simulink model "simulation_base_others"  (R2013a)
settings: Solver=ode4  StartTime=0.0  StopTime=0.2  FixedStep=Ts  RelTol=1e-3
values from neighbouring files (symbols this model uses):
  Cdc = 5e-3    (= 0.005)    [rpg_simulation_base.m]
  Crpcu_each = 1/(2*pi*fs*Zrpcu_each)    [rpg_simulation_base.m]
  ESR = 1e-3    (= 0.001)    [rpg_simulation_base.m]
  fs = 50    [rpg_loss_calculation.m]    (also in rpg_simulation_base.m)
  ftr = 50    [rpg_simulation_base.m]
  Lcable = Xcable/(2*pi*fs)    (= 7.16197243914e-05)    [rpg_simulation_base.m]
  Lload = Xload/wout    [rpg_simulation_base.m]
  Lload1 = Xload1/(2*pi*fs)    [rpg_simulation_base.m]
  Lpri_pu = 0.025    [rpg_simulation_base.m]
  Ls = 1e-3    (= 0.001)    [rpg_simulation_base.m]
  Lsec_pu = 0.025    [rpg_simulation_base.m]
  Ppv = 40e3    (= 40000)    [rpg_simulation_base.m]
  Qpv = 30e3    (= 30000)    [rpg_simulation_base.m]
  Rcable = 56.4e-3    (= 0.0564)    [rpg_simulation_base.m]
  Rload = Zload*pf    [rpg_simulation_base.m]
  Rload1 = Zload1*pfload1    [rpg_simulation_base.m]
  RLs = 10e-3    (= 0.01)    [rpg_simulation_base.m]
  Rpri_pu = 0.0025    [rpg_simulation_base.m]
  Rsec_pu = 0.0025    [rpg_simulation_base.m]
  Rseries = 5    [rpg_simulation_base.m]
  Sbase = 1.6e6    (= 1600000)    [rpg_simulation_base.m]
  Ts = 1e-5    (= 1e-05)    [rpg_simulation_base.m]
  V1 = Vdc*(Rseries+Rrefl)/Rrefl    (= 1083.33333333)    [rpg_simulation_base.m]
  Vdc = 750    [calculate_loss.m]    (also in rpg_loss_calculation.m; rpg_simulation_base.m)
  Vline = 400    [calculate_loss.m]    (also in rpg_loss_calculation.m; rpg_simulation_base.m = 34500)
  Vphase = 400/sqrt(3)    [rpg_simulation_base.m]
  Vpri = 34.5e3    (= 34500)    [rpg_simulation_base.m]
  Vsec = 400    [rpg_simulation_base.m]
  Xs = 2*pi*fs*Ls    (= 0.314159265359)    [rpg_simulation_base.m]
undefined symbols (not defined in the file or in its folder): Lload2, Rload2, rpcu_s1, rpcu_s2, rpcu_s3, rpcu_s4
libraries: powerlib x107, powerlib_meascontrol x18, simulink x1
settings Model: Creator=hp  LastModifiedBy=ugurm

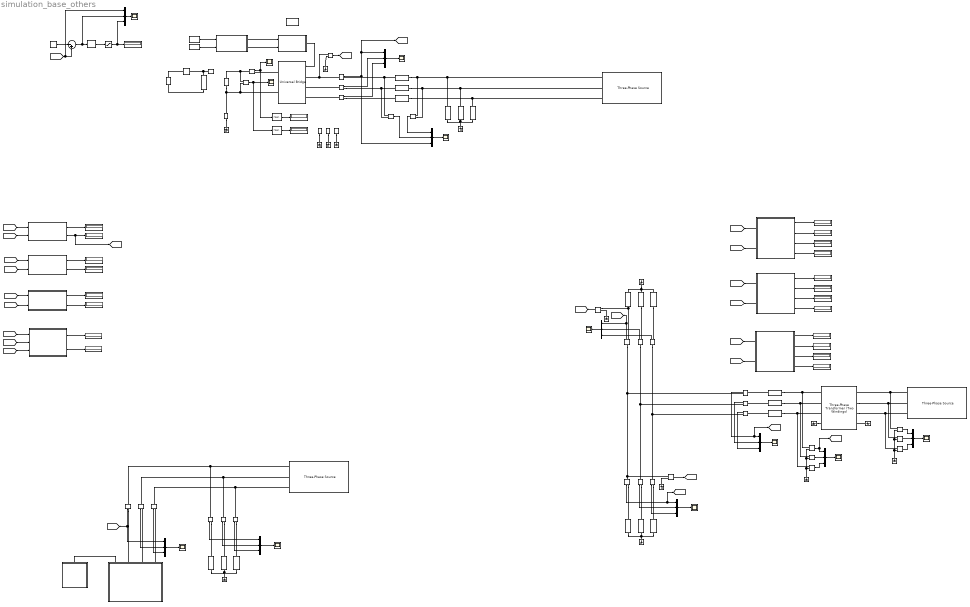
== system simulation_base_others ==
  note: LATER
  note: Grid side P and Q
  note: Load side P and Q
  note: RPCU side P and Q
  note: PV side P and Q
  note: Load-2 P&Q
  note: Load-1 P&Q
  note: PCC P&Q
  Cable_a : powerlib/Elements/Series RLC Branch  LConnTagsString=__new0  RConnTagsString=__new0  BranchType=RL  Resistance=Rcable  Inductance=Lcable  SetiL0=off  InitialCurrent=0  Capacitance=1e-6  Setx0=off  InitialVoltage=0  Measurements=None
  Cable_b : powerlib/Elements/Series RLC Branch  LConnTagsString=__new0  RConnTagsString=__new0  BranchType=RL  Resistance=Rcable  Inductance=Lcable  SetiL0=off  InitialCurrent=0  Capacitance=1e-6  Setx0=off  InitialVoltage=0  Measurements=None
  Cable_c : powerlib/Elements/Series RLC Branch  LConnTagsString=__new0  RConnTagsString=__new0  BranchType=RL  Resistance=Rcable  Inductance=Lcable  SetiL0=off  InitialCurrent=0  Capacitance=1e-6  Setx0=off  InitialVoltage=0  Measurements=None
  Compensation unit : Subsystem
  DC bus cap : powerlib/Elements/Series RLC Branch  LConnTagsString=__new0  RConnTagsString=__new0  BranchType=RC  Resistance=ESR  Inductance=1e-3  SetiL0=off  InitialCurrent=0  Capacitance=Cdc  Setx0=on  InitialVoltage=600  Measurements=None
  Filter_a : powerlib/Elements/Series RLC Branch  LConnTagsString=__new0  RConnTagsString=__new0  BranchType=RL  Resistance=RLs  Inductance=Ls  SetiL0=off  InitialCurrent=0  Capacitance=1e-6  Setx0=off  InitialVoltage=0  Measurements=None
  Filter_b : powerlib/Elements/Series RLC Branch  LConnTagsString=__new0  RConnTagsString=__new0  BranchType=RL  Resistance=RLs  Inductance=Ls  SetiL0=off  InitialCurrent=0  Capacitance=1e-6  Setx0=off  InitialVoltage=0  Measurements=None
  Filter_c : powerlib/Elements/Series RLC Branch  LConnTagsString=__new0  RConnTagsString=__new0  BranchType=RL  Resistance=RLs  Inductance=Ls  SetiL0=off  InitialCurrent=0  Capacitance=1e-6  Setx0=off  InitialVoltage=0  Measurements=None
  Grid (infinite bus) : powerlib/Electrical Sources/Three-Phase Source  Voltage=Vline  PhaseAngle=0  Frequency=fs  InternalConnection=Yg  SpecifyImpedance=off  Resistance=0  Inductance=0  ShortCircuitLevel=100e6  BaseVoltage=Vline  XRratio=7  BusType=swing  Pref=0  Qref=0  Qmin=-inf  Qmax=inf
  Grid (infinite bus)1 : powerlib/Electrical Sources/Three-Phase Source  Voltage=Vline  PhaseAngle=0  Frequency=fs  InternalConnection=Yg  SpecifyImpedance=off  Resistance=1e-9  Inductance=1e-9  ShortCircuitLevel=100e6  BaseVoltage=Vline  XRratio=7  BusType=swing  Pref=0  Qref=0  Qmin=-inf  Qmax=inf
  Grid (infinite bus)2 : powerlib/Electrical Sources/Three-Phase Source  Voltage=400  PhaseAngle=0  Frequency=fs  InternalConnection=Yg  SpecifyImpedance=off  Resistance=0  Inductance=0  ShortCircuitLevel=100e6  BaseVoltage=400  XRratio=7  BusType=swing  Pref=0  Qref=0  Qmin=-inf  Qmax=inf
  Ground{,1..14} (15 alike) : powerlib/Elements/Ground  LConnTagsString=a
  Load_1a : powerlib/Elements/Series RLC Branch  LConnTagsString=__new0  RConnTagsString=__new0  BranchType=RL  Resistance=Rload1  Inductance=Lload1  SetiL0=off  InitialCurrent=0  Capacitance=1e-6  Setx0=off  InitialVoltage=0  Measurements=None
  Load_1b : powerlib/Elements/Series RLC Branch  LConnTagsString=__new0  RConnTagsString=__new0  BranchType=RL  Resistance=Rload1  Inductance=Lload1  SetiL0=off  InitialCurrent=0  Capacitance=1e-6  Setx0=off  InitialVoltage=0  Measurements=None
  Load_1c : powerlib/Elements/Series RLC Branch  LConnTagsString=__new0  RConnTagsString=__new0  BranchType=RL  Resistance=Rload1  Inductance=Lload1  SetiL0=off  InitialCurrent=0  Capacitance=1e-6  Setx0=off  InitialVoltage=0  Measurements=None
  Load_2a : powerlib/Elements/Series RLC Branch  LConnTagsString=__new0  RConnTagsString=__new0  BranchType=RL  Resistance=Rload2  Inductance=Lload2  SetiL0=off  InitialCurrent=0  Capacitance=1e-6  Setx0=off  InitialVoltage=0  Measurements=None
  Load_2a1 : powerlib/Elements/Series RLC Branch  LConnTagsString=__new0  RConnTagsString=__new0  BranchType=RL  Resistance=Rload2  Inductance=Lload2  SetiL0=off  InitialCurrent=0  Capacitance=1e-6  Setx0=off  InitialVoltage=0  Measurements=None
  Load_2a2 : powerlib/Elements/Series RLC Branch  LConnTagsString=__new0  RConnTagsString=__new0  BranchType=RL  Resistance=Rload2  Inductance=Lload2  SetiL0=off  InitialCurrent=0  Capacitance=1e-6  Setx0=off  InitialVoltage=0  Measurements=None
  Load_a1 : powerlib/Elements/Series RLC Branch  LConnTagsString=__new0  RConnTagsString=__new0  BranchType=RL  Resistance=Rload  Inductance=Lload  SetiL0=off  InitialCurrent=0  Capacitance=1e-6  Setx0=off  InitialVoltage=0  Measurements=None
  Load_a2 : powerlib/Elements/Series RLC Branch  LConnTagsString=__new0  RConnTagsString=__new0  BranchType=RL  Resistance=Rload  Inductance=Lload  SetiL0=off  InitialCurrent=0  Capacitance=1e-6  Setx0=off  InitialVoltage=0  Measurements=None
  Load_b1 : powerlib/Elements/Series RLC Branch  LConnTagsString=__new0  RConnTagsString=__new0  BranchType=RL  Resistance=Rload  Inductance=Lload  SetiL0=off  InitialCurrent=0  Capacitance=1e-6  Setx0=off  InitialVoltage=0  Measurements=None
  Load_b2 : powerlib/Elements/Series RLC Branch  LConnTagsString=__new0  RConnTagsString=__new0  BranchType=RL  Resistance=Rload  Inductance=Lload  SetiL0=off  InitialCurrent=0  Capacitance=1e-6  Setx0=off  InitialVoltage=0  Measurements=None
  Load_c1 : powerlib/Elements/Series RLC Branch  LConnTagsString=__new0  RConnTagsString=__new0  BranchType=RL  Resistance=Rload  Inductance=Lload  SetiL0=off  InitialCurrent=0  Capacitance=1e-6  Setx0=off  InitialVoltage=0  Measurements=None
  Load_c2 : powerlib/Elements/Series RLC Branch  LConnTagsString=__new0  RConnTagsString=__new0  BranchType=RL  Resistance=Rload  Inductance=Lload  SetiL0=off  InitialCurrent=0  Capacitance=1e-6  Setx0=off  InitialVoltage=0  Measurements=None
  Mean : powerlib_meascontrol/Measurements/Mean  Freq=1e3  Vinit=0  Ts=0
  Mean1 : powerlib_meascontrol/Measurements/Mean  Freq=1e3  Vinit=0  Ts=0
  Mux{,1..9} (10 alike) : Mux  Inputs=3
  PID Controller : simulink/Continuous/PID Controller  Controller=PID  TimeDomain=Continuous-time  SampleTime=1  IntegratorMethod=Forward Euler  FilterMethod=Forward Euler  Form=Parallel  P=1  I=1  D=0  N=100  InitialConditionSource=internal  InitialConditionForIntegrator=0  InitialConditionForFilter=0  ExternalReset=none  LimitOutput=off  UpperSaturationLimit=inf  LowerSaturationLimit=-inf  LinearizeAsGain=on  AntiWindupMode=none  Kb=1  TrackingMode=off  Kt=1  PParamMin=[]  PParamMax=[]  IParamMin=[]  IParamMax=[]  DParamMin=[]  DParamMax=[]  NParamMin=[]  NParamMax=[]  KbParamMin=[]  KbParamMax=[]  KtParamMin=[]  KtParamMax=[]  POutMin=[]  POutMax=[]  IOutMin=[]  IOutMax=[]  DOutMin=[]  DOutMax=[]  NOutMin=[]  NOutMax=[]  KbOutMin=[]  KbOutMax=[]  KtOutMin=[]  KtOutMax=[]  IntegratorOutMin=[]  IntegratorOutMax=[]  FilterOutMin=[]  FilterOutMax=[]  SumOutMin=[]  SumOutMax=[]  SumI1OutMin=[]  SumI1OutMax=[]  SumI2OutMin=[]  SumI2OutMax=[]  SumI3OutMin=[]  SumI3OutMax=[]  SumDOutMin=[]  SumDOutMax=[]  SaturationOutMin=[]  SaturationOutMax=[]  IntegratorContinuousStateAttributes=''  IntegratorStateMustResolveToSignalObject=off  IntegratorRTWStateStorageClass=Auto  FilterContinuousStateAttributes=''  FilterStateMustResolveToSignalObject=off  FilterRTWStateStorageClass=Auto
  PV_power : Constant  Value=Ppv
  Photovoltaic Inverter : powerlib/Power Electronics/Universal Bridge  Arms=3  SnubberResistance=1e5  SnubberCapacitance=inf  Device=IGBT / Diodes  Ron=1e-3  Lon=0  ForwardVoltages="[  0  0  ]"  ForwardVoltage=0  GTOparameters=[ 10e-6 , 20e-6 ]  IGBTparameters=[ 1e-6 , 2e-6 ]  Measurements=None  Measurements_2=None  converterType=Rectifier
  Pout{,1..22} (23 alike) : Display
      Pout settings: Format=bank
      Pout1 settings: Format=bank
      Pout10 settings: Format=bank
      Pout11 settings: Format=bank
      Pout13 settings: Format=bank
      Pout14 settings: Format=bank
      Pout15 settings: Format=bank
      Pout16 settings: Format=bank
      Pout17 settings: Format=bank
      Pout18 settings: Format=bank
      Pout19 settings: Format=bank
      Pout2 settings: Format=bank
      Pout20 settings: Format=bank
      Pout21 settings: Format=bank
      Pout22 settings: Format=bank
      Pout3 settings: Format=bank
      Pout4 settings: Format=bank
      Pout5 settings: Format=bank
      Pout6 settings: Format=bank
      Pout7 settings: Format=bank
      Pout8 settings: Format=bank
      Pout9 settings: Format=bank
  Pseudo DC Bus : powerlib/Electrical Sources/DC Voltage Source  Amplitude=V1  Measurements=None
  Pseudo DC Bus1 : powerlib/Electrical Sources/DC Voltage Source  Amplitude=Vdc  Measurements=None
  Pseudo res : powerlib/Elements/Series RLC Branch  LConnTagsString=__new0  RConnTagsString=__new0  BranchType=R  Resistance=Rseries  Inductance=1e-3  SetiL0=off  InitialCurrent=0  Capacitance=3e-3  Setx0=off  InitialVoltage=0  Measurements=None
  RPCU kademe ayari : Subsystem
  RP_demand : Constant  Value=Qpv
  Saturation : Saturate  UpperLimit=100000  LowerLimit=0
  Scope{1..12} (12 alike) : Scope
      Scope1 settings: YMin=-175  YMax=225
      Scope10 settings: YMin=-1500  YMax=1500  SaveName=ScopeData10
      Scope11 settings: YMin=-500  YMax=500  SaveName=ScopeData11
      Scope12 settings: YMin=-500  YMax=500  SaveName=ScopeData12
      Scope2 settings: YMin=-30000  YMax=30000  SaveName=ScopeData2
      Scope3 settings: YMin=-500  YMax=500  SaveName=ScopeData3
      Scope4 settings: YMin=-500  YMax=500  SaveName=ScopeData5
      Scope5 settings: YMin=-40  YMax=110
      Scope6 settings: YMin=665  YMax=740  SaveName=ScopeData7
      Scope7 settings: YMin=-800  YMax=800  SaveName=ScopeData6
      Scope8 settings: YMin=-30000  YMax=30000  SaveName=ScopeData8
      Scope9 settings: YMin=74000  YMax=89000  SaveName=ScopeData9
  Sum1 : Sum  Inputs=|-+
  Three-Phase Transformer : powerlib/Elements/Three-Phase Transformer (Two Windings)  Winding1Connection=Yn  UNITS=pu  NominalPower=[Sbase,ftr]  Winding1=[Vpri,Rpri_pu,Lpri_pu]  Winding2Connection=Yn  Winding2=[Vsec,Rsec_pu,Lsec_pu]  SetSaturation=off  Rm=1e6  Lm=1e6  Saturation=[ 0,0 ; 0.0024,1.2 ; 1.0,1.52 ]  Hysteresis=off  DataFile='hysteresis'  SetInitialFlux=off  InitialFluxes=[ 0.8 , -0.8 , 0.7 ]  Measurements=None  MoreParameters=off  BreakLoop=off  DataType=off  TransfoNumber=1
  earth{,1..3} (4 alike) : powerlib/Elements/Series RLC Branch  LConnTagsString=__new0  RConnTagsString=__new0  BranchType=R  Resistance=1e12  Inductance=Lload  SetiL0=off  InitialCurrent=0  Capacitance=1e-6  Setx0=off  InitialVoltage=0  Measurements=None
  grid_rp* : Constant  Value=0
  ia : powerlib/Measurements/Current Measurement  PhasorSimulation=off  OutputType=Complex  PSBequivalent=0
  ia_grid : powerlib/Measurements/Current Measurement  PhasorSimulation=off  OutputType=Complex  PSBequivalent=0
  ia_load : powerlib/Measurements/Current Measurement  PhasorSimulation=off  OutputType=Complex  PSBequivalent=0
  ia_load1 : powerlib/Measurements/Current Measurement  PhasorSimulation=off  OutputType=Complex  PSBequivalent=0
  ia_load2 : powerlib/Measurements/Current Measurement  PhasorSimulation=off  OutputType=Complex  PSBequivalent=0
  ia_rpcu : powerlib/Measurements/Current Measurement  PhasorSimulation=off  OutputType=Complex  PSBequivalent=0
  ib : powerlib/Measurements/Current Measurement  PhasorSimulation=off  OutputType=Complex  PSBequivalent=0
  ib_grid : powerlib/Measurements/Current Measurement  PhasorSimulation=off  OutputType=Complex  PSBequivalent=0
  ib_load{,1..3} (4 alike) : powerlib/Measurements/Current Measurement  PhasorSimulation=off  OutputType=Complex  PSBequivalent=0
  ib_rpcu : powerlib/Measurements/Current Measurement  PhasorSimulation=off  OutputType=Complex  PSBequivalent=0
  ic : powerlib/Measurements/Current Measurement  PhasorSimulation=off  OutputType=Complex  PSBequivalent=0
  ic_grid : powerlib/Measurements/Current Measurement  PhasorSimulation=off  OutputType=Complex  PSBequivalent=0
  ic_load : powerlib/Measurements/Current Measurement  PhasorSimulation=off  OutputType=Complex  PSBequivalent=0
  ic_load1 : powerlib/Measurements/Current Measurement  PhasorSimulation=off  OutputType=Complex  PSBequivalent=0
  ic_rpcu : powerlib/Measurements/Current Measurement  PhasorSimulation=off  OutputType=Complex  PSBequivalent=0
  idc : powerlib/Measurements/Current Measurement  PhasorSimulation=off  OutputType=Complex  PSBequivalent=0
  measure1_grid : Subsystem
  measure1_grid1 : Subsystem
  measure1_grid2 : Subsystem
  measure1_grid3 : Subsystem
  measure1_grid4 : Subsystem
  measure2_load : Subsystem
  measure2_rpcu : Subsystem
  powergui : powerlib/powergui  Priority=1  SimulationMode=Discrete  SolverType=Tustin  SampleTime=Ts  frequency=60  SPID=off  DisableSnubberDevices=off  DisableRonSwitches=off  DisableVfSwitches=off  SwTol=0  Interpol=off  DisplayEquations=off  frequencyindice=50  Pbase=100e6  ErrMax=1e-4  Iterations=50  UnitsV=kV  UnitsW=MW  FunctionMessages=off  echomessages=off  HookPort=off  EnableUseOfTLC=off  x0status=blocks  RestoreLinks=warning  ResistiveCurrentMeasurement=off  Frange=[0:2:500]  Ylog=off  Xlog=on  ShowGrid=off  save=off  variable=ZData  ZoomFFT=off  StartTime=0.0  cycles=1  DisplayStyle=1  fundamental=60  FreqAxis=off  MaxFrequency=1000  frequencyindicesteady=1  RmsSteady=1  display=off  Ts=0  methode=off
  pv control : Subsystem
  pw pwm : Subsystem
  ser : powerlib/Elements/Series RLC Branch  LConnTagsString=__new0  RConnTagsString=__new0  BranchType=R  Resistance=1e-6  Inductance=Lload  SetiL0=off  InitialCurrent=0  Capacitance=1e-6  Setx0=off  InitialVoltage=0  Measurements=None
  vdc : powerlib/Measurements/Voltage Measurement  PhasorSimulation=off  OutputType=Complex  PSBequivalent=0
  vsa{,1..10} (11 alike) : powerlib/Measurements/Voltage Measurement  PhasorSimulation=off  OutputType=Complex  PSBequivalent=0
  tag scope: Iload1=global, Iload2=global, Ipcc=global, Ipv_a=global, Irpcu_a=global, Vc_a=global, Vload1=global, Vload2=global, Vpcc=global, grid_rp=global
  wires:
  RPCU kademe ayari/1(kademe) -> Compensation unit/1(Kademe)
  ib/1 -> Mux/2
  ic/1 -> Mux/3
  Mux/1 -> Scope1/1
  pw pwm/1(gate1) -> Photovoltaic Inverter/1
  Mux1/1 -> Scope2/1
  ib_rpcu/1 -> Mux1/2
  ic_rpcu/1 -> Mux1/3
  Mux2/1 -> Scope3/1
  ia_load/1 -> [Iload1], Mux2/1
  ib_load/1 -> Mux2/2
  ic_load/1 -> Mux2/3
  Mux3/1 -> Scope4/1
  ib_grid/1 -> Mux3/2
  ic_grid/1 -> Mux3/3
  ia_grid/1 -> [Ipcc], Mux3/1
  vdc/1 -> Mean1/1, Scope6/1
  [Vpcc_a] -> measure2_load/1(Va)
  [Vpcc_a] -> measure1_grid/1(Va)
  [Igrid_a] -> measure1_grid/2(Ia)
  [Iload_a] -> measure2_load/2(Ia)
  [Vpcc_a] -> measure2_rpcu/1(Va)
  [Irpcu_a] -> measure2_rpcu/2(Ia)
  ia_rpcu/1 -> [Irpcu_a], Mux1/1
  measure1_grid/1(Pm1) -> Pout/1
  measure2_load/1(Pm2) -> Pout1/1
  measure2_rpcu/1(Pm3) -> Pout2/1
  measure1_grid/2(Qm1) -> [grid_rp], Pout3/1
  measure2_load/2(Qm2) -> Pout4/1
  measure2_rpcu/2(Qm3) -> Pout5/1
  idc/1 -> Scope5/1, Mean/1
  Mean/1 -> Pout6/1
  Mean1/1 -> Pout7/1
  Mux4/1 -> Scope7/1
  vsa2/1 -> Mux4/1
  vsa1/1 -> Mux4/2
  ia/1 -> Mux4/3, [Ipv_a], Mux/1
  vsa3/1 -> [Vc_a]
  [Vpcc_a] -> measure1_grid1/1(Va)
  [Ipv_a] -> measure1_grid1/2(Ia)
  measure1_grid1/1(Pm1) -> Pout8/1
  measure1_grid1/2(Qm1) -> Pout9/1
  [Vc_a] -> measure1_grid1/3(Vpv)
  grid_rp*/1 -> Sum1/1
  [grid_rp] -> Sum1/2, Mux5/1
  Sum1/1 -> Mux5/2, PID Controller/1
  PID Controller/1 -> Saturation/1
  PV_power/1 -> pv control/2(Ppv)
  Saturation/1 -> Pout12/1, Mux5/3
  Mux5/1 -> Scope9/1
  pv control/1(ma) -> pw pwm/1(ma)
  pv control/2(delta) -> pw pwm/2(delta)
  RP_demand/1 -> pv control/1(Qpv)
  Mux6/1 -> Scope8/1
  vsa5/1 -> Mux6/2
  vsa6/1 -> Mux6/3
  vsa4/1 -> Mux6/1
  Mux7/1 -> Scope10/1
  vsa8/1 -> Mux7/2
  vsa9/1 -> Mux7/3
  vsa7/1 -> Mux7/1, [Vpcc]
  Mux9/1 -> Scope12/1
  ia_load1/1 -> Mux9/1
  ib_load1/1 -> Mux9/2
  ic_load1/1 -> Mux9/3
  ib_load3/1 -> Mux8/3
  ib_load2/1 -> Mux8/2
  ia_load2/1 -> [Iload2], Mux8/1
  Mux8/1 -> Scope11/1
  vsa/1 -> [Vload2]
  vsa10/1 -> [Vload1]
  [Vpcc] -> measure1_grid4/1(Va)
  [Ipcc] -> measure1_grid4/2(Ia)
  measure1_grid4/1(Pm1) -> Pout15/1
  measure1_grid4/2(Qm1) -> Pout16/1
  measure1_grid4/3(Vrms) -> Pout19/1
  measure1_grid4/4(powerf) -> Pout20/1
  [Vload2] -> measure1_grid3/1(Va)
  [Iload2] -> measure1_grid3/2(Ia)
  [Vload1] -> measure1_grid2/1(Va)
  [Iload1] -> measure1_grid2/2(Ia)
  measure1_grid2/1(Pm1) -> Pout10/1
  measure1_grid2/2(Qm1) -> Pout11/1
  measure1_grid2/3(Vrms) -> Pout13/1
  measure1_grid2/4(powerf) -> Pout14/1
  measure1_grid3/1(Pm1) -> Pout17/1
  measure1_grid3/2(Qm1) -> Pout18/1
  measure1_grid3/3(Vrms) -> Pout21/1
  measure1_grid3/4(powerf) -> Pout22/1
  connections:
  Photovoltaic Inverter/RConn2 -- Pseudo DC Bus1/LConn1 -- earth/LConn1 -- vdc/LConn2
  Pseudo res/RConn1 -- Pseudo DC Bus/RConn1
  DC bus cap/LConn1 -- ser/RConn1 -- Pseudo res/LConn1
  ia/LConn1 -- vsa3/LConn1 -- Photovoltaic Inverter/LConn1
  Filter_a/LConn1 -- ia/RConn1 -- vsa1/LConn1
  ib/LConn1 -- Photovoltaic Inverter/LConn2
  ib/RConn1 -- vsa1/LConn2 -- Filter_b/LConn1
  ic/LConn1 -- Photovoltaic Inverter/LConn3
  ic/RConn1 -- Filter_c/LConn1
  ia_load/RConn1 -- Load_1a/LConn1
  ic_load/RConn1 -- Load_1c/LConn1
  ib_load/RConn1 -- Load_1b/LConn1
  Ground/LConn1 -- Load_1a/RConn1 -- Load_1c/RConn1 -- Load_1b/RConn1
  Ground1/LConn1 -- vsa/LConn2
  ic_load/LConn1 -- ib_load3/LConn1 -- ic_grid/RConn1
  ib_load/LConn1 -- ib_load2/LConn1 -- ib_grid/RConn1
  ia_load/LConn1 -- ia_grid/RConn1 -- ia_load2/LConn1 -- vsa10/LConn1
  Compensation unit/LConn2 -- ib_rpcu/RConn1
  Compensation unit/LConn3 -- ic_rpcu/RConn1
  ia_rpcu/RConn1 -- Compensation unit/LConn1
  vsa2/LConn1 -- Filter_a/RConn1 -- Load_a1/LConn1 -- Grid (infinite bus)1/RConn1
  vsa2/LConn2 -- Grid (infinite bus)1/RConn2 -- Load_b1/LConn1 -- Filter_b/RConn1
  vdc/LConn1 -- Pseudo DC Bus1/RConn1 -- idc/LConn1
  Photovoltaic Inverter/RConn1 -- idc/RConn1
  earth/RConn1 -- Ground2/LConn1
  earth1/RConn1 -- Ground3/LConn1
  earth2/RConn1 -- Ground4/LConn1
  earth3/RConn1 -- Ground5/LConn1
  Ground6/LConn1 -- vsa3/LConn2
  Load_b1/RConn1 -- Load_a1/RConn1 -- Ground7/LConn1 -- Load_c1/RConn1
  DC bus cap/RConn1 -- Pseudo DC Bus/LConn1
  Filter_c/RConn1 -- Grid (infinite bus)1/RConn3 -- Load_c1/LConn1
  Three-Phase Transformer/RConn1 -- Cable_a/RConn1 -- vsa7/LConn1
  Three-Phase Transformer/RConn2 -- Cable_b/RConn1 -- vsa8/LConn1
  Three-Phase Transformer/RConn3 -- Cable_c/RConn1 -- vsa9/LConn1
  Grid (infinite bus)/RConn1 -- vsa4/LConn1 -- Three-Phase Transformer/LConn1
  Three-Phase Transformer/LConn2 -- vsa5/LConn1 -- Grid (infinite bus)/RConn2
  Three-Phase Transformer/LConn3 -- vsa6/LConn1 -- Grid (infinite bus)/RConn3
  Ground8/LConn1 -- vsa6/LConn2 -- vsa4/LConn2 -- vsa5/LConn2
  Cable_a/LConn1 -- ia_grid/LConn1
  Cable_b/LConn1 -- ib_grid/LConn1
  Cable_c/LConn1 -- ic_grid/LConn1
  Ground9/LConn1 -- vsa9/LConn2 -- vsa7/LConn2 -- vsa8/LConn2
  Ground11/LConn1 -- Three-Phase Transformer/LConn4
  Ground10/LConn1 -- Three-Phase Transformer/RConn4
  Grid (infinite bus)2/RConn3 -- ic_load1/LConn1 -- ic_rpcu/LConn1
  Grid (infinite bus)2/RConn2 -- ib_rpcu/LConn1 -- ib_load1/LConn1
  Grid (infinite bus)2/RConn1 -- ia_load1/LConn1 -- ia_rpcu/LConn1
  Load_b2/RConn1 -- Ground13/LConn1 -- Load_a2/RConn1 -- Load_c2/RConn1
  ia_load1/RConn1 -- Load_a2/LConn1
  ic_load1/RConn1 -- Load_c2/LConn1
  ib_load1/RConn1 -- Load_b2/LConn1
  Ground12/LConn1 -- Load_2a2/RConn1 -- Load_2a1/RConn1 -- Load_2a/RConn1
  Load_2a/LConn1 -- ia_load2/RConn1 -- vsa/LConn1
  Load_2a1/LConn1 -- ib_load2/RConn1
  Load_2a2/LConn1 -- ib_load3/RConn1
  Ground14/LConn1 -- vsa10/LConn2

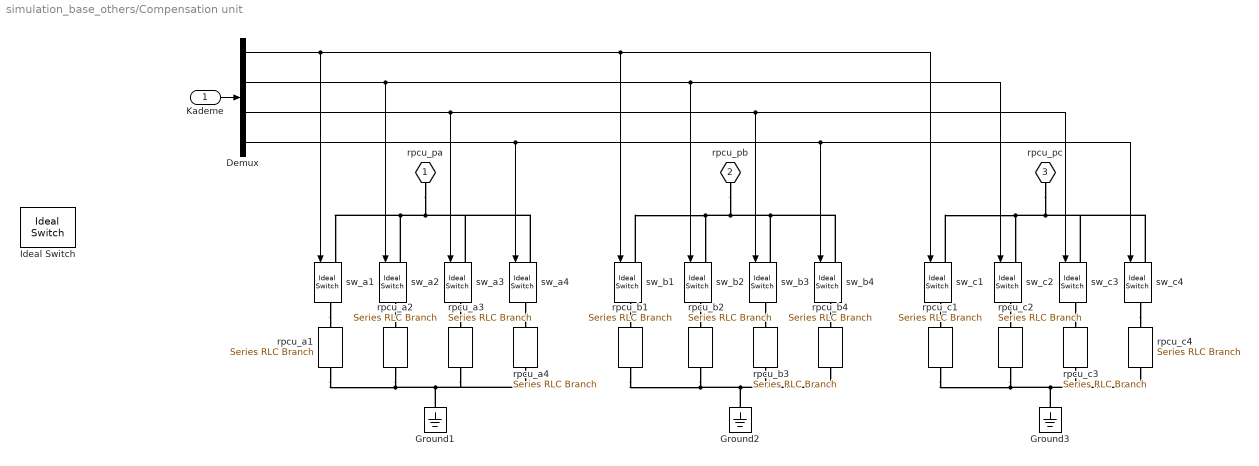
== system simulation_base_others/Compensation unit ==
  Kademe : Inport
  " sw_a2" : powerlib/Power Electronics/Ideal Switch  Ron=0.001  Lon=0  IC=0  Rs=1e5  Cs=inf  Measurements=off
  Demux : Demux
  Ground1 : powerlib/Elements/Ground  LConnTagsString=a
  Ground2 : powerlib/Elements/Ground  LConnTagsString=a
  Ground3 : powerlib/Elements/Ground  LConnTagsString=a
  Ideal Switch : powerlib/Power Electronics/Ideal Switch  Ron=0.001  Lon=0  IC=0  Rs=1e5  Cs=inf  Measurements=on
  rpcu_a{1..4} (4 alike) : powerlib/Elements/Series RLC Branch  LConnTagsString=__new0  RConnTagsString=__new0  BranchType=C  Resistance=1e9  Inductance=1e-6  SetiL0=off  InitialCurrent=0  Capacitance=Crpcu_each  Setx0=off  InitialVoltage=0  Measurements=None
  rpcu_b{1..4} (4 alike) : powerlib/Elements/Series RLC Branch  LConnTagsString=__new0  RConnTagsString=__new0  BranchType=C  Resistance=1e9  Inductance=1e-6  SetiL0=off  InitialCurrent=0  Capacitance=Crpcu_each  Setx0=off  InitialVoltage=0  Measurements=None
  rpcu_c{1..4} (4 alike) : powerlib/Elements/Series RLC Branch  LConnTagsString=__new0  RConnTagsString=__new0  BranchType=C  Resistance=1e9  Inductance=1e-6  SetiL0=off  InitialCurrent=0  Capacitance=Crpcu_each  Setx0=off  InitialVoltage=0  Measurements=None
  sw_a1 : powerlib/Power Electronics/Ideal Switch  Ron=0.001  Lon=0  IC=0  Rs=1e5  Cs=inf  Measurements=off
  sw_a3 : powerlib/Power Electronics/Ideal Switch  Ron=0.001  Lon=0  IC=0  Rs=1e5  Cs=inf  Measurements=off
  sw_a4 : powerlib/Power Electronics/Ideal Switch  Ron=0.001  Lon=0  IC=0  Rs=1e5  Cs=inf  Measurements=off
  sw_b{1..4} (4 alike) : powerlib/Power Electronics/Ideal Switch  Ron=1e-9  Lon=0  IC=0  Rs=1e12  Cs=inf  Measurements=off
  sw_c{1..4} (4 alike) : powerlib/Power Electronics/Ideal Switch  Ron=1e-9  Lon=0  IC=0  Rs=1e12  Cs=inf  Measurements=off
  rpcu_pa : PMIOPort  Port=1  Side=Left
  rpcu_pb : PMIOPort  Port=2  Side=Left
  rpcu_pc : PMIOPort  Port=3  Side=Left
  wires:
  Kademe/1 -> Demux/1
  Demux/1 -> sw_c1/1, sw_b1/1, sw_a1/1
  Demux/2 -> sw_b2/1, sw_c2/1, " sw_a2"/1
  Demux/3 -> sw_c3/1, sw_b3/1, sw_a3/1
  Demux/4 -> sw_c4/1, sw_b4/1, sw_a4/1
  connections:
  Ground1/LConn1 -- rpcu_a2/RConn1 -- rpcu_a1/RConn1 -- rpcu_a4/RConn1 -- rpcu_a3/RConn1
  " sw_a2"/LConn1 -- rpcu_pa/RConn1 -- sw_a3/LConn1 -- sw_a4/LConn1 -- sw_a1/LConn1
  sw_a3/RConn1 -- rpcu_a3/LConn1
  " sw_a2"/RConn1 -- rpcu_a2/LConn1
  sw_a4/RConn1 -- rpcu_a4/LConn1
  rpcu_b1/RConn1 -- rpcu_b4/RConn1 -- rpcu_b3/RConn1 -- Ground2/LConn1 -- rpcu_b2/RConn1
  sw_b4/LConn1 -- sw_b3/LConn1 -- rpcu_pb/RConn1 -- sw_b2/LConn1 -- sw_b1/LConn1
  sw_b1/RConn1 -- rpcu_b1/LConn1
  sw_b4/RConn1 -- rpcu_b4/LConn1
  sw_b3/RConn1 -- rpcu_b3/LConn1
  sw_b2/RConn1 -- rpcu_b2/LConn1
  sw_c3/RConn1 -- rpcu_c3/LConn1
  sw_c1/RConn1 -- rpcu_c1/LConn1
  sw_c4/RConn1 -- rpcu_c4/LConn1
  sw_c2/RConn1 -- rpcu_c2/LConn1
  sw_c1/LConn1 -- rpcu_pc/RConn1 -- sw_c3/LConn1 -- sw_c4/LConn1 -- sw_c2/LConn1
  rpcu_c1/RConn1 -- rpcu_c2/RConn1 -- Ground3/LConn1 -- rpcu_c4/RConn1 -- rpcu_c3/RConn1
  sw_a1/RConn1 -- rpcu_a1/LConn1

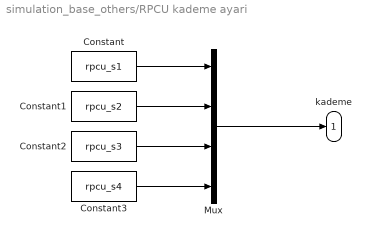
== system simulation_base_others/RPCU kademe ayari ==
  Constant : Constant  Value=rpcu_s1
  Constant1 : Constant  Value=rpcu_s2
  Constant2 : Constant  Value=rpcu_s3
  Constant3 : Constant  Value=rpcu_s4
  Mux : Mux
  kademe : Outport
  wires:
  Constant1/1 -> Mux/2
  Constant/1 -> Mux/1
  Mux/1 -> kademe/1
  Constant3/1 -> Mux/4
  Constant2/1 -> Mux/3

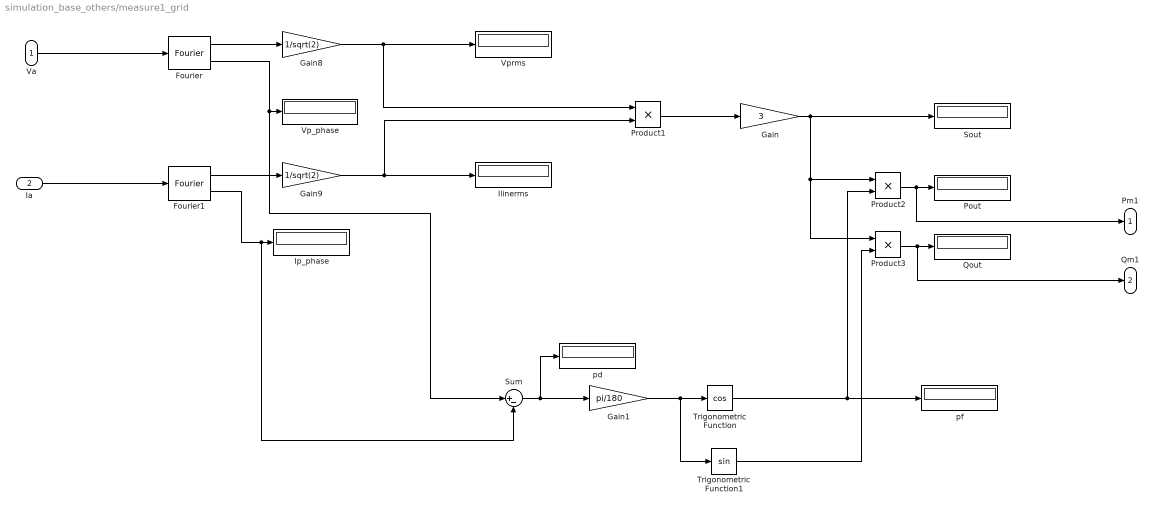
== system simulation_base_others/measure1_grid ==
  Va : Inport
  Ia : Inport  Port=2
  Fourier : powerlib_meascontrol/Measurements/Fourier  Freq=50  n=1  InInit=[0, 0]  Ts=0
  Fourier1 : powerlib_meascontrol/Measurements/Fourier  Freq=50  n=1  InInit=[0, 0]  Ts=0
  Gain : Gain  Gain=3
  Gain1 : Gain  Gain=pi/180
  Gain8 : Gain  Gain=1/sqrt(2)
  Gain9 : Gain  Gain=1/sqrt(2)
  "Ilinerms " : Display
  Ip_phase : Display
  Pout : Display
  Product1 : Product
  Product2 : Product
  Product3 : Product
  Qout : Display
  Sout : Display
      settings: Format=short_e
  Sum : Sum  Inputs=|+-
  Trigonometric Function : Trigonometry  Operator=cos
  Trigonometric Function1 : Trigonometry
  Vp_phase : Display
  "Vprms " : Display
  pd : Display
  pf : Display
  Pm1 : Outport
  Qm1 : Outport  Port=2
  wires:
  Gain8/1 -> "Vprms "/1, Product1/1
  Ia/1 -> Fourier1/1
  Fourier1/1 -> Gain9/1
  Va/1 -> Fourier/1
  Fourier/1 -> Gain8/1
  Product1/1 -> Gain/1
  Gain/1 -> Sout/1, Product2/1, Product3/1
  Trigonometric Function/1 -> pf/1, Product2/2
  Gain1/1 -> Trigonometric Function1/1, Trigonometric Function/1
  Product2/1 -> Pm1/1, Pout/1
  Fourier/2 -> Sum/1, Vp_phase/1
  Gain9/1 -> "Ilinerms "/1, Product1/2
  Fourier1/2 -> Sum/2, Ip_phase/1
  Sum/1 -> Gain1/1, pd/1
  Trigonometric Function1/1 -> Product3/2
  Product3/1 -> Qm1/1, Qout/1

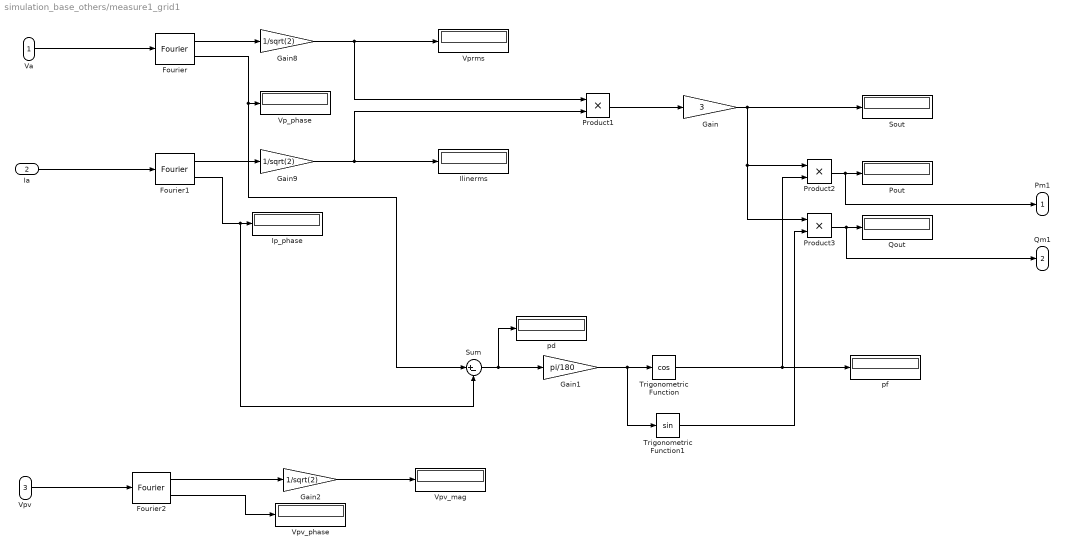
== system simulation_base_others/measure1_grid1 ==
  Va : Inport
  Ia : Inport  Port=2
  Vpv : Inport  Port=3
  Fourier : powerlib_meascontrol/Measurements/Fourier  Freq=50  n=1  InInit=[0, 0]  Ts=0
  Fourier1 : powerlib_meascontrol/Measurements/Fourier  Freq=50  n=1  InInit=[0, 0]  Ts=0
  Fourier2 : powerlib_meascontrol/Measurements/Fourier  Freq=50  n=1  InInit=[0, 0]  Ts=0
  Gain : Gain  Gain=3
  Gain1 : Gain  Gain=pi/180
  Gain2 : Gain  Gain=1/sqrt(2)
  Gain8 : Gain  Gain=1/sqrt(2)
  Gain9 : Gain  Gain=1/sqrt(2)
  "Ilinerms " : Display
  Ip_phase : Display
  Pout : Display
  Product1 : Product
  Product2 : Product
  Product3 : Product
  Qout : Display
  Sout : Display
      settings: Format=short_e
  Sum : Sum  Inputs=|+-
  Trigonometric Function : Trigonometry  Operator=cos
  Trigonometric Function1 : Trigonometry
  Vp_phase : Display
  "Vprms " : Display
  Vpv_mag : Display
  Vpv_phase : Display
  pd : Display
  pf : Display
  Pm1 : Outport
  Qm1 : Outport  Port=2
  wires:
  Gain8/1 -> "Vprms "/1, Product1/1
  Ia/1 -> Fourier1/1
  Fourier1/1 -> Gain9/1
  Va/1 -> Fourier/1
  Fourier/1 -> Gain8/1
  Product1/1 -> Gain/1
  Gain/1 -> Sout/1, Product2/1, Product3/1
  Trigonometric Function/1 -> pf/1, Product2/2
  Gain1/1 -> Trigonometric Function1/1, Trigonometric Function/1
  Product2/1 -> Pm1/1, Pout/1
  Fourier/2 -> Sum/1, Vp_phase/1
  Gain9/1 -> "Ilinerms "/1, Product1/2
  Fourier1/2 -> Sum/2, Ip_phase/1
  Sum/1 -> Gain1/1, pd/1
  Trigonometric Function1/1 -> Product3/2
  Product3/1 -> Qm1/1, Qout/1
  Fourier2/1 -> Gain2/1
  Fourier2/2 -> Vpv_phase/1
  Gain2/1 -> Vpv_mag/1
  Vpv/1 -> Fourier2/1

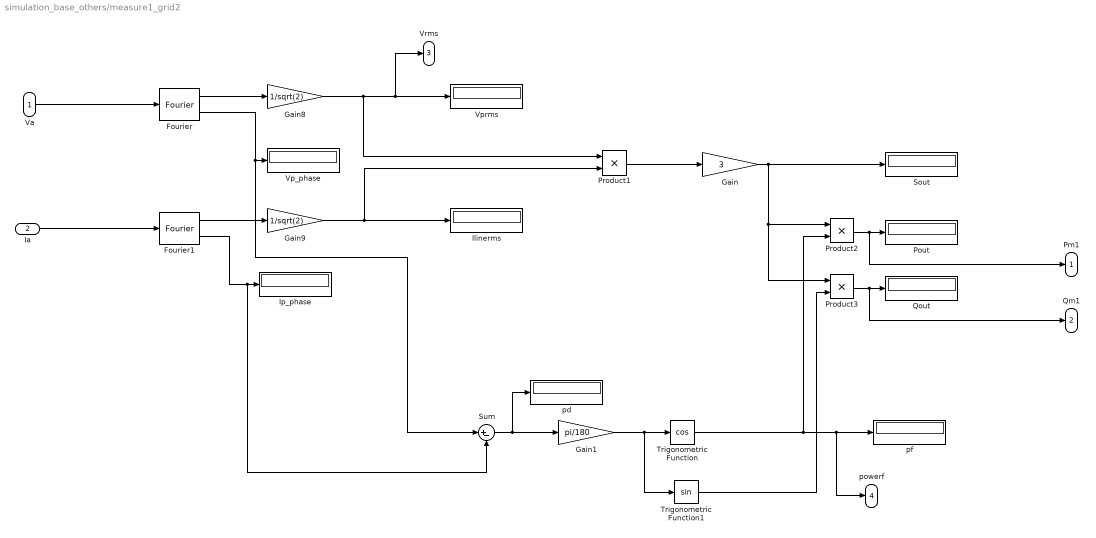
== system simulation_base_others/measure1_grid2 ==
  Va : Inport
  Ia : Inport  Port=2
  Fourier : powerlib_meascontrol/Measurements/Fourier  Freq=50  n=1  InInit=[0, 0]  Ts=0
  Fourier1 : powerlib_meascontrol/Measurements/Fourier  Freq=50  n=1  InInit=[0, 0]  Ts=0
  Gain : Gain  Gain=3
  Gain1 : Gain  Gain=pi/180
  Gain8 : Gain  Gain=1/sqrt(2)
  Gain9 : Gain  Gain=1/sqrt(2)
  "Ilinerms " : Display
  Ip_phase : Display
  Pout : Display
  Product1 : Product
  Product2 : Product
  Product3 : Product
  Qout : Display
  Sout : Display
      settings: Format=short_e
  Sum : Sum  Inputs=|+-
  Trigonometric Function : Trigonometry  Operator=cos
  Trigonometric Function1 : Trigonometry
  Vp_phase : Display
  "Vprms " : Display
  pd : Display
  pf : Display
  Pm1 : Outport
  Qm1 : Outport  Port=2
  Vrms : Outport  Port=3
  powerf : Outport  Port=4
  wires:
  Gain8/1 -> Vrms/1, "Vprms "/1, Product1/1
  Ia/1 -> Fourier1/1
  Fourier1/1 -> Gain9/1
  Va/1 -> Fourier/1
  Fourier/1 -> Gain8/1
  Product1/1 -> Gain/1
  Gain/1 -> Sout/1, Product2/1, Product3/1
  Trigonometric Function/1 -> powerf/1, pf/1, Product2/2
  Gain1/1 -> Trigonometric Function1/1, Trigonometric Function/1
  Product2/1 -> Pm1/1, Pout/1
  Fourier/2 -> Sum/1, Vp_phase/1
  Gain9/1 -> "Ilinerms "/1, Product1/2
  Fourier1/2 -> Sum/2, Ip_phase/1
  Sum/1 -> Gain1/1, pd/1
  Trigonometric Function1/1 -> Product3/2
  Product3/1 -> Qm1/1, Qout/1

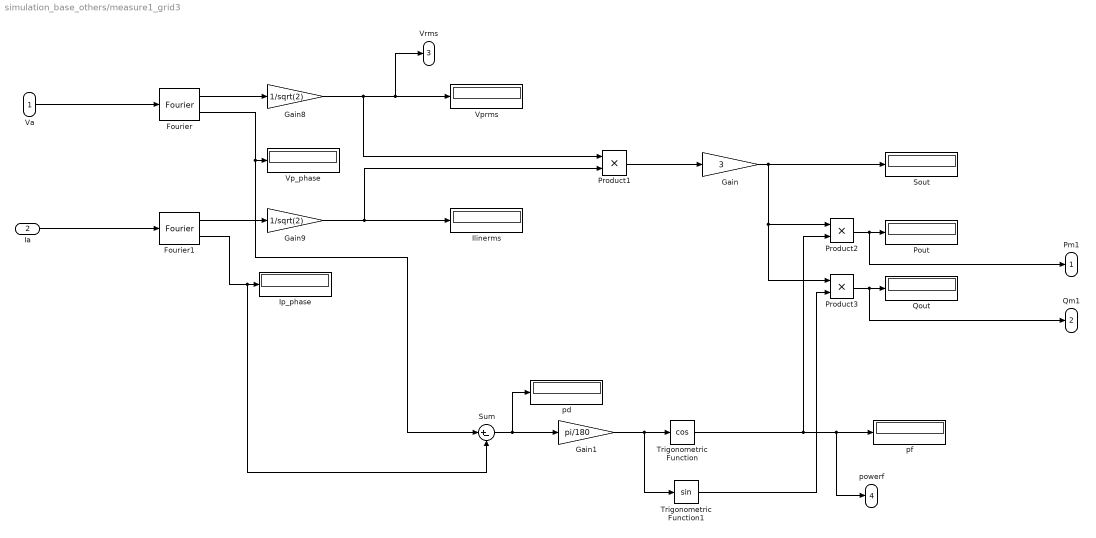
== system simulation_base_others/measure1_grid3 ==
  Va : Inport
  Ia : Inport  Port=2
  Fourier : powerlib_meascontrol/Measurements/Fourier  Freq=50  n=1  InInit=[0, 0]  Ts=0
  Fourier1 : powerlib_meascontrol/Measurements/Fourier  Freq=50  n=1  InInit=[0, 0]  Ts=0
  Gain : Gain  Gain=3
  Gain1 : Gain  Gain=pi/180
  Gain8 : Gain  Gain=1/sqrt(2)
  Gain9 : Gain  Gain=1/sqrt(2)
  "Ilinerms " : Display
  Ip_phase : Display
  Pout : Display
  Product1 : Product
  Product2 : Product
  Product3 : Product
  Qout : Display
  Sout : Display
      settings: Format=short_e
  Sum : Sum  Inputs=|+-
  Trigonometric Function : Trigonometry  Operator=cos
  Trigonometric Function1 : Trigonometry
  Vp_phase : Display
  "Vprms " : Display
  pd : Display
  pf : Display
  Pm1 : Outport
  Qm1 : Outport  Port=2
  Vrms : Outport  Port=3
  powerf : Outport  Port=4
  wires:
  Gain8/1 -> Vrms/1, "Vprms "/1, Product1/1
  Ia/1 -> Fourier1/1
  Fourier1/1 -> Gain9/1
  Va/1 -> Fourier/1
  Fourier/1 -> Gain8/1
  Product1/1 -> Gain/1
  Gain/1 -> Sout/1, Product2/1, Product3/1
  Trigonometric Function/1 -> powerf/1, pf/1, Product2/2
  Gain1/1 -> Trigonometric Function1/1, Trigonometric Function/1
  Product2/1 -> Pm1/1, Pout/1
  Fourier/2 -> Sum/1, Vp_phase/1
  Gain9/1 -> "Ilinerms "/1, Product1/2
  Fourier1/2 -> Sum/2, Ip_phase/1
  Sum/1 -> Gain1/1, pd/1
  Trigonometric Function1/1 -> Product3/2
  Product3/1 -> Qm1/1, Qout/1

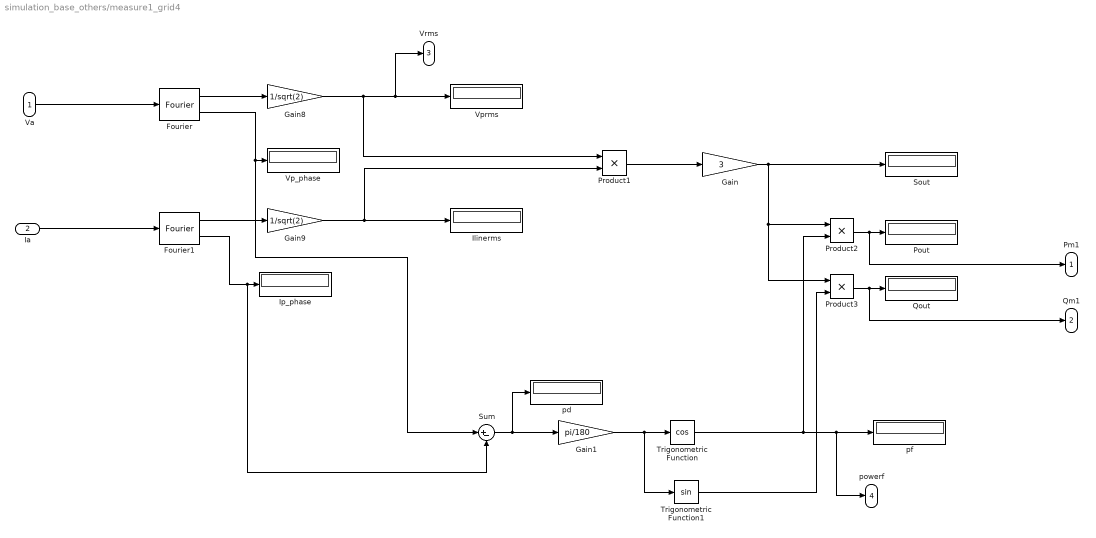
== system simulation_base_others/measure1_grid4 ==
  Va : Inport
  Ia : Inport  Port=2
  Fourier : powerlib_meascontrol/Measurements/Fourier  Freq=50  n=1  InInit=[0, 0]  Ts=0
  Fourier1 : powerlib_meascontrol/Measurements/Fourier  Freq=50  n=1  InInit=[0, 0]  Ts=0
  Gain : Gain  Gain=3
  Gain1 : Gain  Gain=pi/180
  Gain8 : Gain  Gain=1/sqrt(2)
  Gain9 : Gain  Gain=1/sqrt(2)
  "Ilinerms " : Display
  Ip_phase : Display
  Pout : Display
  Product1 : Product
  Product2 : Product
  Product3 : Product
  Qout : Display
  Sout : Display
      settings: Format=short_e
  Sum : Sum  Inputs=|+-
  Trigonometric Function : Trigonometry  Operator=cos
  Trigonometric Function1 : Trigonometry
  Vp_phase : Display
  "Vprms " : Display
  pd : Display
  pf : Display
  Pm1 : Outport
  Qm1 : Outport  Port=2
  Vrms : Outport  Port=3
  powerf : Outport  Port=4
  wires:
  Gain8/1 -> Vrms/1, "Vprms "/1, Product1/1
  Ia/1 -> Fourier1/1
  Fourier1/1 -> Gain9/1
  Va/1 -> Fourier/1
  Fourier/1 -> Gain8/1
  Product1/1 -> Gain/1
  Gain/1 -> Sout/1, Product2/1, Product3/1
  Trigonometric Function/1 -> powerf/1, pf/1, Product2/2
  Gain1/1 -> Trigonometric Function1/1, Trigonometric Function/1
  Product2/1 -> Pm1/1, Pout/1
  Fourier/2 -> Sum/1, Vp_phase/1
  Gain9/1 -> "Ilinerms "/1, Product1/2
  Fourier1/2 -> Sum/2, Ip_phase/1
  Sum/1 -> Gain1/1, pd/1
  Trigonometric Function1/1 -> Product3/2
  Product3/1 -> Qm1/1, Qout/1

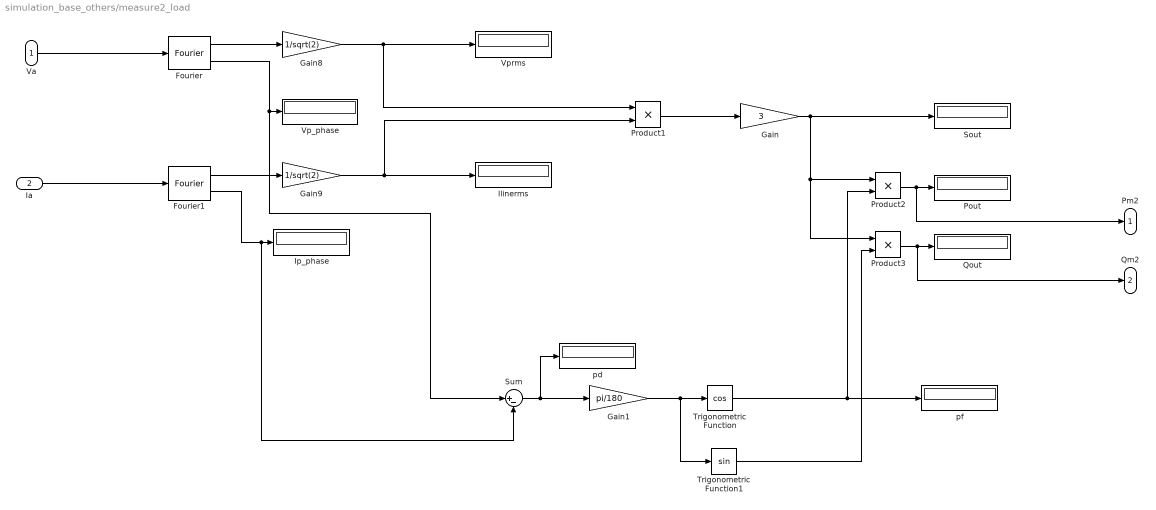
== system simulation_base_others/measure2_load ==
  Va : Inport
  Ia : Inport  Port=2
  Fourier : powerlib_meascontrol/Measurements/Fourier  Freq=50  n=1  InInit=[0, 0]  Ts=0
  Fourier1 : powerlib_meascontrol/Measurements/Fourier  Freq=50  n=1  InInit=[0, 0]  Ts=0
  Gain : Gain  Gain=3
  Gain1 : Gain  Gain=pi/180
  Gain8 : Gain  Gain=1/sqrt(2)
  Gain9 : Gain  Gain=1/sqrt(2)
  "Ilinerms " : Display
  Ip_phase : Display
  Pout : Display
  Product1 : Product
  Product2 : Product
  Product3 : Product
  Qout : Display
  Sout : Display
      settings: Format=short_e
  Sum : Sum  Inputs=|+-
  Trigonometric Function : Trigonometry  Operator=cos
  Trigonometric Function1 : Trigonometry
  Vp_phase : Display
  "Vprms " : Display
  pd : Display
  pf : Display
  Pm2 : Outport
  Qm2 : Outport  Port=2
  wires:
  Gain8/1 -> "Vprms "/1, Product1/1
  Ia/1 -> Fourier1/1
  Fourier1/1 -> Gain9/1
  Va/1 -> Fourier/1
  Fourier/1 -> Gain8/1
  Product1/1 -> Gain/1
  Gain/1 -> Sout/1, Product2/1, Product3/1
  Trigonometric Function/1 -> pf/1, Product2/2
  Gain1/1 -> Trigonometric Function1/1, Trigonometric Function/1
  Product2/1 -> Pm2/1, Pout/1
  Fourier/2 -> Sum/1, Vp_phase/1
  Gain9/1 -> "Ilinerms "/1, Product1/2
  Fourier1/2 -> Sum/2, Ip_phase/1
  Sum/1 -> Gain1/1, pd/1
  Trigonometric Function1/1 -> Product3/2
  Product3/1 -> Qm2/1, Qout/1

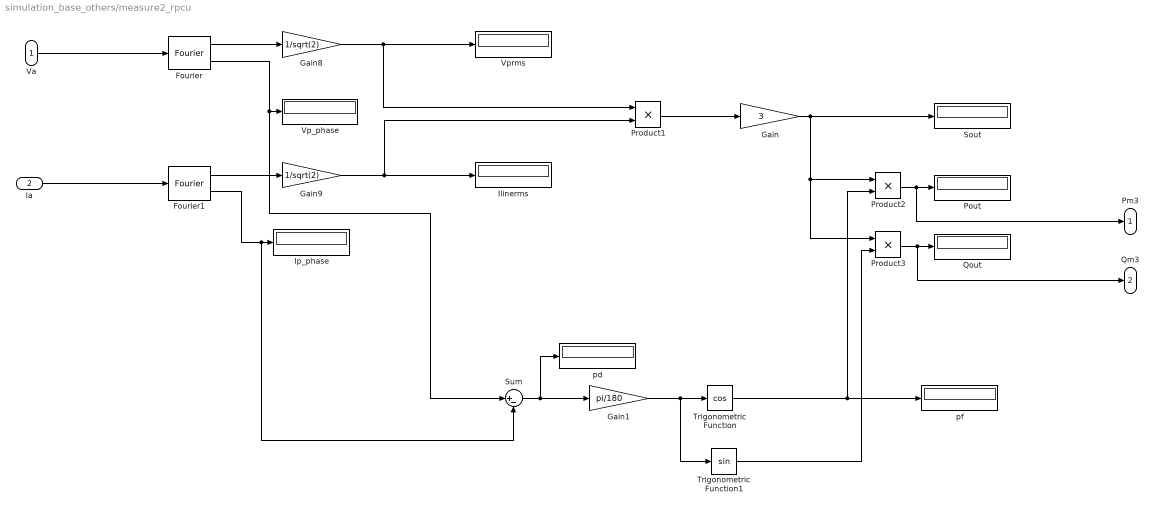
== system simulation_base_others/measure2_rpcu ==
  Va : Inport
  Ia : Inport  Port=2
  Fourier : powerlib_meascontrol/Measurements/Fourier  Freq=50  n=1  InInit=[0, 0]  Ts=0
  Fourier1 : powerlib_meascontrol/Measurements/Fourier  Freq=50  n=1  InInit=[0, 0]  Ts=0
  Gain : Gain  Gain=3
  Gain1 : Gain  Gain=pi/180
  Gain8 : Gain  Gain=1/sqrt(2)
  Gain9 : Gain  Gain=1/sqrt(2)
  "Ilinerms " : Display
  Ip_phase : Display
  Pout : Display
  Product1 : Product
  Product2 : Product
  Product3 : Product
  Qout : Display
  Sout : Display
      settings: Format=short_e
  Sum : Sum  Inputs=|+-
  Trigonometric Function : Trigonometry  Operator=cos
  Trigonometric Function1 : Trigonometry
  Vp_phase : Display
  "Vprms " : Display
  pd : Display
  pf : Display
  Pm3 : Outport
  Qm3 : Outport  Port=2
  wires:
  Gain8/1 -> "Vprms "/1, Product1/1
  Ia/1 -> Fourier1/1
  Fourier1/1 -> Gain9/1
  Va/1 -> Fourier/1
  Fourier/1 -> Gain8/1
  Product1/1 -> Gain/1
  Gain/1 -> Sout/1, Product2/1, Product3/1
  Trigonometric Function/1 -> pf/1, Product2/2
  Gain1/1 -> Trigonometric Function1/1, Trigonometric Function/1
  Product2/1 -> Pm3/1, Pout/1
  Fourier/2 -> Sum/1, Vp_phase/1
  Gain9/1 -> "Ilinerms "/1, Product1/2
  Fourier1/2 -> Sum/2, Ip_phase/1
  Sum/1 -> Gain1/1, pd/1
  Trigonometric Function1/1 -> Product3/2
  Product3/1 -> Qm3/1, Qout/1

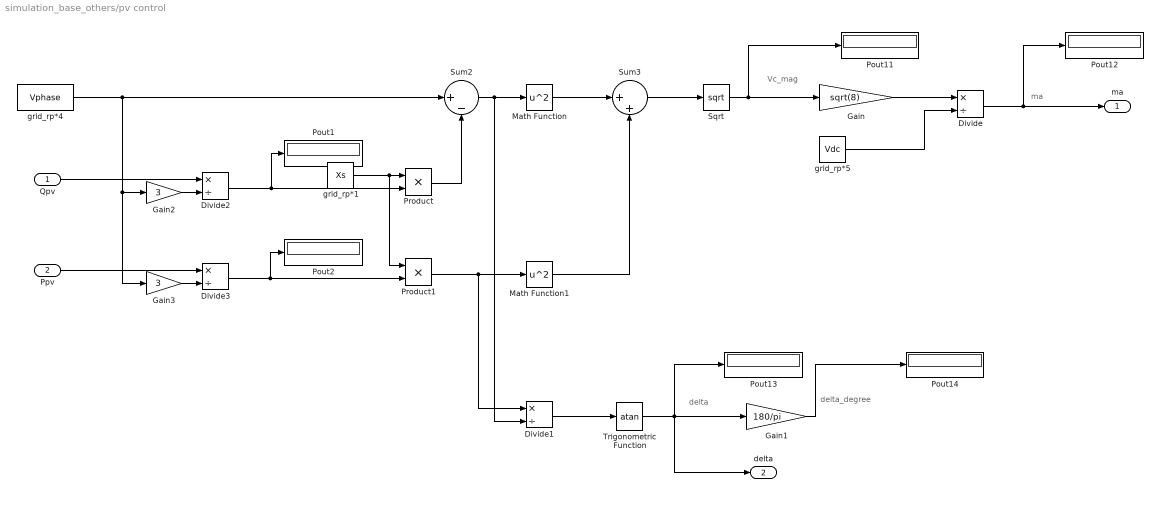
== system simulation_base_others/pv control ==
  note: delta_degree
  note: delta
  note: ma
  note: Vc_mag
  Qpv : Inport
  Ppv : Inport  Port=2
  Divide{,1..3} (4 alike) : Product  Inputs=*/
  Gain : Gain  Gain=sqrt(8)
  Gain1 : Gain  Gain=180/pi
  Gain2 : Gain  Gain=3
  Gain3 : Gain  Gain=3
  Math Function : Math  Operator=square  SaturateOnIntegerOverflow=on
  Math Function1 : Math  Operator=square  SaturateOnIntegerOverflow=on
  Pout{1..2,11..14} (6 alike) : Display
      Pout11 settings: Format=bank
  Product : Product
  Product1 : Product
  Sqrt : Sqrt  SaturateOnIntegerOverflow=on
  Sum2 : Sum  Inputs=|+-
  Sum3 : Sum  Inputs=|++
  Trigonometric Function : Trigonometry  Operator=atan  OutputSignalType=real
  grid_rp*1 : Constant  Value=Xs
  grid_rp*4 : Constant  Value=Vphase
  grid_rp*5 : Constant  Value=Vdc
  ma : Outport
  delta : Outport  Port=2
  wires:
  Product1/1 -> Divide1/1, Math Function1/1
  Divide2/1 -> Pout1/1, Product/2
  Gain/1 -> Divide/1
  Divide3/1 -> Pout2/1, Product1/2
  Product/1 -> Sum2/2
  Gain1/1 -> Pout14/1
  Sqrt/1 -> Gain/1, Pout11/1
  Math Function/1 -> Sum3/1
  Math Function1/1 -> Sum3/2
  Sum3/1 -> Sqrt/1
  Sum2/1 -> Divide1/2, Math Function/1
  grid_rp*5/1 -> Divide/2
  Trigonometric Function/1 -> delta/1, Pout13/1, Gain1/1
  Divide/1 -> ma/1, Pout12/1
  Divide1/1 -> Trigonometric Function/1
  grid_rp*1/1 -> Product1/1, Product/1
  Qpv/1 -> Divide2/1
  Gain2/1 -> Divide2/2
  grid_rp*4/1 -> Gain3/1, Gain2/1, Sum2/1
  Ppv/1 -> Divide3/1
  Gain3/1 -> Divide3/2

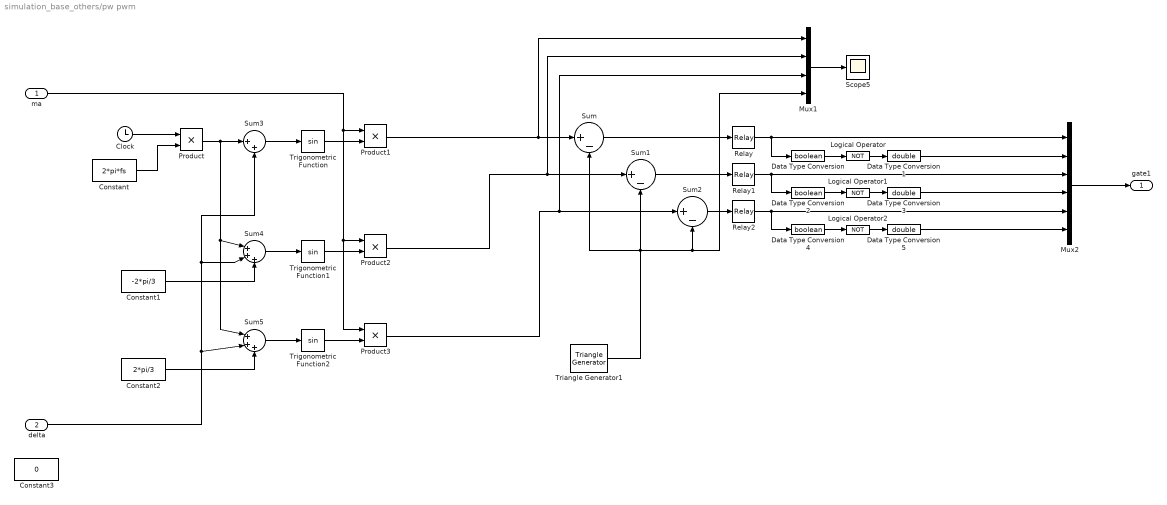
== system simulation_base_others/pw pwm ==
  ma : Inport
  delta : Inport  Port=2
  Clock : Clock
  Constant : Constant  Value=2*pi*fs
  Constant1 : Constant  Value=-2*pi/3
  Constant2 : Constant  Value=2*pi/3
  Constant3 : Constant  Value=0
  Data Type Conversion : DataTypeConversion  OutDataTypeStr=boolean
  Data Type Conversion1 : DataTypeConversion  OutDataTypeStr=double
  Data Type Conversion2 : DataTypeConversion  OutDataTypeStr=boolean
  Data Type Conversion3 : DataTypeConversion  OutDataTypeStr=double
  Data Type Conversion4 : DataTypeConversion  OutDataTypeStr=boolean
  Data Type Conversion5 : DataTypeConversion  OutDataTypeStr=double
  Logical Operator : Logic  Operator=NOT  AllPortsSameDT=off  OutDataTypeStr=boolean
  Logical Operator1 : Logic  Operator=NOT  AllPortsSameDT=off  OutDataTypeStr=boolean
  Logical Operator2 : Logic  Operator=NOT  AllPortsSameDT=off  OutDataTypeStr=boolean
  Mux1 : Mux
  Mux2 : Mux  Inputs=6
  Product{,1..3} (4 alike) : Product
  Relay : Relay
  Relay1 : Relay
  Relay2 : Relay
  Scope5 : Scope
      settings: YMin=-2  YMax=2  SaveName=ScopeData4
  Sum : Sum  Inputs=|+-
  Sum1 : Sum  Inputs=|+-
  Sum2 : Sum  Inputs=|+-
  Sum3 : Sum  Inputs=|++
  Sum4 : Sum  Inputs=|+++
  Sum5 : Sum  Inputs=|+++
  Triangle Generator1 : powerlib_meascontrol/Pulse & Signal Generators/Triangle Generator  Freq=fsw  Phase=0  Ts=0
  Trigonometric Function : Trigonometry
  Trigonometric Function1 : Trigonometry
  Trigonometric Function2 : Trigonometry
  gate1 : Outport
  wires:
  Triangle Generator1/1 -> Mux1/4, Sum2/2, Sum1/2, Sum/2
  Product2/1 -> Mux1/2, Sum1/1
  Product3/1 -> Mux1/3, Sum2/1
  Sum/1 -> Relay/1
  Sum1/1 -> Relay1/1
  Sum2/1 -> Relay2/1
  Data Type Conversion/1 -> Logical Operator/1
  Relay/1 -> Data Type Conversion/1, Mux2/1
  Logical Operator/1 -> Data Type Conversion1/1
  Data Type Conversion1/1 -> Mux2/2
  Data Type Conversion2/1 -> Logical Operator1/1
  Relay1/1 -> Data Type Conversion2/1, Mux2/3
  Logical Operator1/1 -> Data Type Conversion3/1
  Data Type Conversion3/1 -> Mux2/4
  Data Type Conversion4/1 -> Logical Operator2/1
  Relay2/1 -> Data Type Conversion4/1, Mux2/5
  Logical Operator2/1 -> Data Type Conversion5/1
  Mux2/1 -> gate1/1
  Data Type Conversion5/1 -> Mux2/6
  Clock/1 -> Product/1
  Constant/1 -> Product/2
  Sum3/1 -> Trigonometric Function/1
  Trigonometric Function/1 -> Product1/2
  Constant1/1 -> Sum4/3
  Sum4/1 -> Trigonometric Function1/1
  Trigonometric Function1/1 -> Product2/2
  Product/1 -> Sum5/1, Sum4/1, Sum3/1
  delta/1 -> Sum3/2, Sum4/2, Sum5/2
  ma/1 -> Product3/1, Product2/1, Product1/1
  Constant2/1 -> Sum5/3
  Sum5/1 -> Trigonometric Function2/1
  Trigonometric Function2/1 -> Product3/2
  Product1/1 -> Mux1/1, Sum/1
  Mux1/1 -> Scope5/1
